simulink subsystem "PieroControladoV"  (R2023b)
settings: Solver=VariableStepAuto  StartTime=0.0  StopTime=10.0  RelTol=1e-3
settings Model: Creator=Usuario_UMA  LastModifiedBy=Daniel

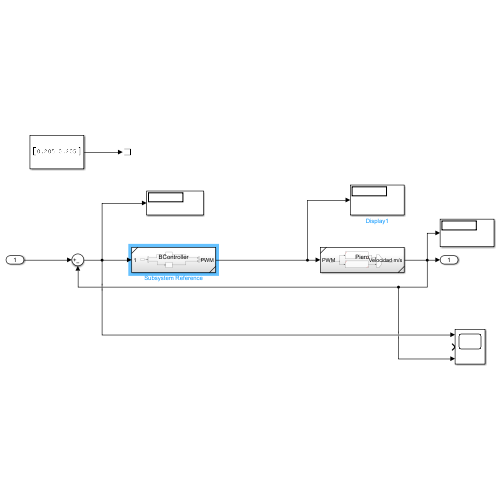
[thumbnail: Simulink's stored preview of the top-level diagram]
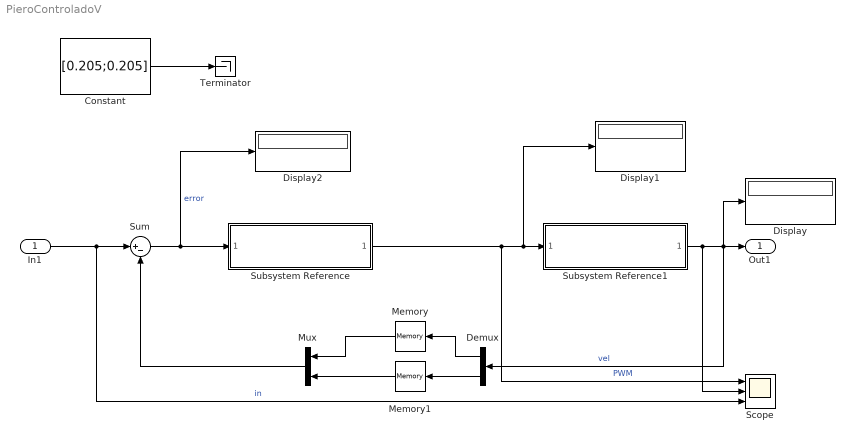
== system PieroControladoV ==
  In1 : Inport
  Constant : Constant  Value=[0.205;0.205]
  Demux : Demux  Outputs=2
  Display : Display
  Display1 : Display
  Display2 : Display
  Memory : Memory
  Memory1 : Memory
  Mux : Mux  Inputs=2
  Scope : Scope  NumInputPorts=3
  Subsystem Reference : Subsystem  ReferencedSubsystem=BController
  Subsystem Reference1 : Subsystem  ReferencedSubsystem=Piero
  Sum : Sum  Inputs=|+-
  Terminator : Terminator
  Out1 : Outport
  wires:
  Sum/1 -> Subsystem Reference/1, Display2/1  "error"
  Subsystem Reference/1 -> Subsystem Reference1/1, Display1/1, Scope/1  "PWM"
  Subsystem Reference1/1 -> Out1/1, Display/1, Demux/1, Scope/2  "vel"
  In1/1 -> Sum/1, Scope/3  "in"
  Constant/1 -> Terminator/1
  Demux/2 -> Memory1/1
  Demux/1 -> Memory/1
  Memory/1 -> Mux/1
  Memory1/1 -> Mux/2
  Mux/1 -> Sum/2
